simulink model "open_loop"  (R2019a)
settings: Solver=FixedStepAuto  StartTime=0.0  StopTime=10.0  FixedStep=1/100  RelTol=1e-3  AbsTol=1e-3
model workspace: external: MATLAB File params.m (data not in the file)
values from neighbouring files (symbols this model uses):
  An = double(subs(A, [x;ctrl] , [x_lin; u_lin] ))    [linearization.m]
  b = 2.75E-11    (= 2.75e-11)    [linearization.m]    (also in main.m)
  Bn = double(subs(B, [x;ctrl] , [x_lin; u_lin] ))    [linearization.m]
  Cn = eye(size(x,1))    [linearization.m]
  Dn = zeros(size(x,1),4)    [linearization.m]
  g = 9.81    [linearization.m]    (also in main.m)
  k = 1E-9    (= 1e-09)    [linearization.m]    (also in main.m)
  m = 0.027    [linearization.m]    (also in main.m)
  scenario = 1    [main.m]
  u_lin = repmat(0.027*g/4, [4 1])    [main.m]
  x0 = [0 0 0  0 0 0  deg2rad(20) deg2rad(20) deg2rad(0) 0 0 0]'    [main.m]
  x_lin = zeros(12,1)    [main.m]
undefined symbols (not defined in the file or in its folder): sigbuilder_block
libraries: nesl_utility x9
settings Model: Creator=Jocke  LastModifiedBy=lucas
settings SolverCC: AutoScaleAbsTol=off
settings DataIOCC: ReturnWorkspaceOutputs=off
settings DebuggingCC: ArithmeticOperatorsInVariantConditions=warning
settings SFSimCC: SimUseLocalCustomCode=off
settings RTWCC: RTWUseLocalCustomCode=off
settings CodeAppCC: StateflowObjectComments=on
settings SimscapeCC: SimscapeNormalizeSystem=off  SimscapeLogType=all  SimscapeLogDataHistory=10000

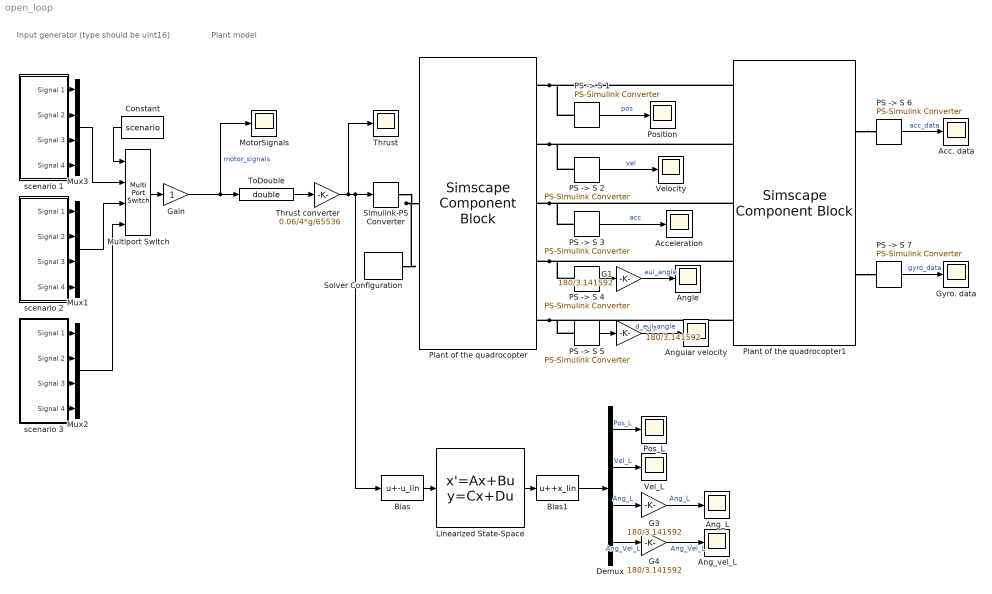
== system open_loop ==
  note: Input generator
      | (type should be uint16)
  note: Plant model
  Acc. data : Scope
  Acceleration : Scope
  Ang_L : Scope
  Ang_vel_L : Scope
  Angle : Scope
  Angular velocity : Scope
  Bias : Bias  Bias=-u_lin
  Bias1 : Bias  Bias=+x_lin
  Constant : Constant  Value=scenario
  Demux : Demux
  G{1..4} (4 alike) : Gain  Gain=180/3.141592
  Gain : Gain
  Gyro. data : Scope
  Linearized State-Space : StateSpace  A=An  B=Bn  C=Cn  D=Dn  InitialCondition=x0
  MotorSignals : Scope
  Multiport Switch : MultiPortSwitch
  Mux1 : Mux
  Mux2 : Mux
  Mux3 : Mux
  PS -> S {1..7} (7 alike) : nesl_utility/PS-Simulink Converter  PhysicalDomain=network_engine_domain  SubClassName=ps_output  LeftPortType=input  RightPortType=output  PseudoPeriodic=off  Frequencies=[]  Unit=1  AffineConversion=off
  Plant of the quadrocopter : SimscapeComponentBlock  SourceFile=plant  ComponentPath=plant  ComponentVariants=plant  ComponentVariantNames=plant  ClassName=plant  SchemaVersion=1  m=m kg  g=g m/s^2  d=d m  k=k s^2*N/rad^2  b=b N*m/(rad/s)^2
      settings: CopyFcn=simscape.engine.sli.internal.componentblockcallback(gcbh,'COPY')  PreCopyFcn=simscape.engine.sli.internal.componentblockcallback(gcbh,'PRECOPY')  PreDeleteFcn=simscape.engine.sli.internal.componentblockcallback(gcbh,'PREDELETE')
      mask Type: Plant of quadrocopter
  Plant of the quadrocopter1 : SimscapeComponentBlock  SourceFile=sensors  ComponentPath=sensors  ComponentVariants=sensors  ComponentVariantNames=sensors  ClassName=sensors  SchemaVersion=1  m=m kg  g=g m/s^2  d=d m  k=k  b=b
      settings: CopyFcn=simscape.engine.sli.internal.componentblockcallback(gcbh,'COPY')  PreCopyFcn=simscape.engine.sli.internal.componentblockcallback(gcbh,'PRECOPY')  PreDeleteFcn=simscape.engine.sli.internal.componentblockcallback(gcbh,'PREDELETE')
      mask Type: Plant of quadrocopter
  Pos_L : Scope
  Position : Scope
  Simulink-PS Converter : nesl_utility/Simulink-PS Converter  PhysicalDomain=network_engine_domain  SubClassName=ps_input  LeftPortType=input  RightPortType=output  PseudoPeriodic=off  Frequencies=[]  NoiseDistribution=none  NoiseParameters=[]  Unit=1  AffineConversion=off  FilteringAndDerivatives=zero  SimscapeFilterOrder=1  InputFilterTimeConstant=0.001  UdotUserProvided=1
  Solver Configuration : nesl_utility/Solver Configuration  PhysicalDomain=network_engine_domain  SubClassName=solver  LeftPortType=input  RightPortType=generic  Tones=[]  Harmonics=[]  SimulateNoise=off  Profile=off  UseLocalSampling=off  EnableSwitchedLinearOptims=on  FrequencyDomain=off  UseCCode=off  RelTol=0.001  AbsTol=1e-06  MinStep=1e-09  ToWorkspace=off  RevertToSquareIcSolve=off  NumHomotopyIterations=100  PhasorMode=off  PhasorModeNumHarmonics=1  DoDC=off  ResidualTolerance=1e-09  UseLocalSolver=off  LocalSolverChoice=NE_BACKWARD_EULER_ADVANCER  LocalSolverSampleTime=0.001  DoFixedCost=off  MaxNonlinIter=3  MaxModeIter=2  LinearAlgebra=Sparse  EquationFormulation=NE_TIME_EF  DelaysMemoryBudget=1024  AutomaticFiltering=on  FilteringTimeConstant=0.001  PartitionStorageMethod=AS_NEEDED  PartitionMemoryBudget=1024  PartitionMethod=FAST
  Thrust : Scope
  Thrust converter : Gain  Gain=0.06/4*g/65536
  ToDouble : DataTypeConversion  OutDataTypeStr=double  RndMeth=Round  SaturateOnIntegerOverflow=on
  Vel_L : Scope
  Velocity : Scope
  scenario 1 : Subsystem  Tag=STV Subsys  LoadFcn=sigbuilder_block('load');  StartFcn=sigbuilder_block('start');  StopFcn=sigbuilder_block('stop');  ClipboardFcn=sigbuilder_block('clipboard');  mask(Sigbuilder block){tuvar=[0:10]}
      mask help: Simulink:masks:SigbuilderBlock_MD
      mask init:
      | if ~strcmp(get_param(bdroot(gcbh),'SimulationStatus'),'stopped') tuvar = sigbuilder_block('maskInit'); end
      settings: CopyFcn=sigbuilder_block('copy');  DeleteFcn=sigbuilder_block('delete');  ModelCloseFcn=sigbuilder_block('modelClose');  PreSaveFcn=sigbuilder_block('preSave');  PauseFcn=sigbuilder_block('pause');  ContinueFcn=sigbuilder_block('continue');  NameChangeFcn=sigbuilder_block('namechange');  OpenFcn=sigbuilder_block('open',[382.5 57 795 560.25 ]);  CloseFcn=sigbuilder_block('close');
      mask Display: plot(0, 0, 100, 100,[2, 2, 32, 32, 2], [68, 8, 8, 68, 68],[32, 2], [38, 38], [32, 19, 2],[53, 60, 44], [32, 17, 17, 2],[16, 16, 31, 31]);txt = getActiveGroup(gcbh);text(2, 100, txt,'verticalAlignment', 'top');
  scenario 2 : Subsystem  Tag=STV Subsys  LoadFcn=sigbuilder_block('load');  StartFcn=sigbuilder_block('start');  StopFcn=sigbuilder_block('stop');  ClipboardFcn=sigbuilder_block('clipboard');  mask(Sigbuilder block){tuvar=[0:10]}
      mask help: Simulink:masks:SigbuilderBlock_MD
      mask init:
      | if ~strcmp(get_param(bdroot(gcbh),'SimulationStatus'),'stopped') tuvar = sigbuilder_block('maskInit'); end
      settings: CopyFcn=sigbuilder_block('copy');  DeleteFcn=sigbuilder_block('delete');  ModelCloseFcn=sigbuilder_block('modelClose');  PreSaveFcn=sigbuilder_block('preSave');  PauseFcn=sigbuilder_block('pause');  ContinueFcn=sigbuilder_block('continue');  NameChangeFcn=sigbuilder_block('namechange');  OpenFcn=sigbuilder_block('open',[378.75 53.25 795 560.25 ]);  CloseFcn=sigbuilder_block('close');
      mask Display: plot(0, 0, 100, 100,[2, 2, 32, 32, 2], [68, 8, 8, 68, 68],[32, 2], [38, 38], [32, 19, 2],[53, 60, 44], [32, 17, 17, 2],[16, 16, 31, 31]);txt = getActiveGroup(gcbh);text(2, 100, txt,'verticalAlignment', 'top');
  scenario 3 : Subsystem  Tag=STV Subsys  LoadFcn=sigbuilder_block('load');  StartFcn=sigbuilder_block('start');  StopFcn=sigbuilder_block('stop');  ClipboardFcn=sigbuilder_block('clipboard');  mask(Sigbuilder block){tuvar=[0:10]}
      mask help: Simulink:masks:SigbuilderBlock_MD
      mask init:
      | if ~strcmp(get_param(bdroot(gcbh),'SimulationStatus'),'stopped') tuvar = sigbuilder_block('maskInit'); end
      settings: CopyFcn=sigbuilder_block('copy');  DeleteFcn=sigbuilder_block('delete');  ModelCloseFcn=sigbuilder_block('modelClose');  PreSaveFcn=sigbuilder_block('preSave');  PauseFcn=sigbuilder_block('pause');  ContinueFcn=sigbuilder_block('continue');  NameChangeFcn=sigbuilder_block('namechange');  OpenFcn=sigbuilder_block('open',[285.75 75.75 817.5 560.25 ]);  CloseFcn=sigbuilder_block('close');
      mask Display: plot(0, 0, 100, 100,[2, 2, 32, 32, 2], [68, 8, 8, 68, 68],[32, 2], [38, 38], [32, 19, 2],[53, 60, 44], [32, 17, 17, 2],[16, 16, 31, 31]);txt = getActiveGroup(gcbh);text(2, 100, txt,'verticalAlignment', 'top');
  wires:
  "PS -> S 7"/1 -> Gyro. data/1  "gyro_data"
  "PS -> S 6"/1 -> Acc. data/1  "acc_data"
  Multiport Switch/1 -> Gain/1
  G1/1 -> Angle/1  "eul_angle"
  G2/1 -> Angular velocity/1  "d_eul_angle"
  ToDouble/1 -> Thrust converter/1
  Thrust converter/1 -> Bias/1, Simulink-PS Converter/1, Thrust/1
  "PS -> S 1"/1 -> Position/1  "pos"
  "PS -> S 5"/1 -> G2/1
  "PS -> S 4"/1 -> G1/1
  "PS -> S 3"/1 -> Acceleration/1  "acc"
  "PS -> S 2"/1 -> Velocity/1  "vel"
  scenario 1/2(Signal 2) -> Mux3/2
  scenario 1/1(Signal 1) -> Mux3/1
  scenario 1/3(Signal 3) -> Mux3/3
  scenario 1/4(Signal 4) -> Mux3/4
  scenario 2/3(Signal 3) -> Mux1/3
  scenario 2/4(Signal 4) -> Mux1/4
  scenario 2/2(Signal 2) -> Mux1/2
  Mux1/1 -> Multiport Switch/3
  scenario 2/1(Signal 1) -> Mux1/1
  Mux3/1 -> Multiport Switch/2
  Gain/1 -> MotorSignals/1, ToDouble/1  "motor_signals"
  scenario 3/3(Signal 3) -> Mux2/3
  scenario 3/4(Signal 4) -> Mux2/4
  scenario 3/2(Signal 2) -> Mux2/2
  scenario 3/1(Signal 1) -> Mux2/1
  Mux2/1 -> Multiport Switch/4
  Constant/1 -> Multiport Switch/1
  Linearized State-Space/1 -> Bias1/1
  Demux/1 -> Pos_L/1  "Pos_L"
  Demux/2 -> Vel_L/1  "Vel_L"
  Bias/1 -> Linearized State-Space/1
  Bias1/1 -> Demux/1
  G3/1 -> Ang_L/1  "Ang_L"
  Demux/3 -> G3/1  "Ang_L"
  G4/1 -> Ang_vel_L/1  "Ang_Vel_L"
  Demux/4 -> G4/1  "Ang_Vel_L"
  connections:
  Plant of the quadrocopter/LConn1 -- Solver Configuration/RConn1 -- Simulink-PS Converter/RConn1
  Plant of the quadrocopter/RConn1 -- "PS -> S 1"/LConn1 -- Plant of the quadrocopter1/LConn1
  Plant of the quadrocopter/RConn2 -- "PS -> S 2"/LConn1 -- Plant of the quadrocopter1/LConn2
  Plant of the quadrocopter/RConn3 -- "PS -> S 3"/LConn1 -- Plant of the quadrocopter1/LConn3
  Plant of the quadrocopter/RConn4 -- "PS -> S 4"/LConn1 -- Plant of the quadrocopter1/LConn4
  Plant of the quadrocopter/RConn5 -- "PS -> S 5"/LConn1 -- Plant of the quadrocopter1/LConn5
  Plant of the quadrocopter1/RConn1 -- "PS -> S 6"/LConn1
  Plant of the quadrocopter1/RConn2 -- "PS -> S 7"/LConn1

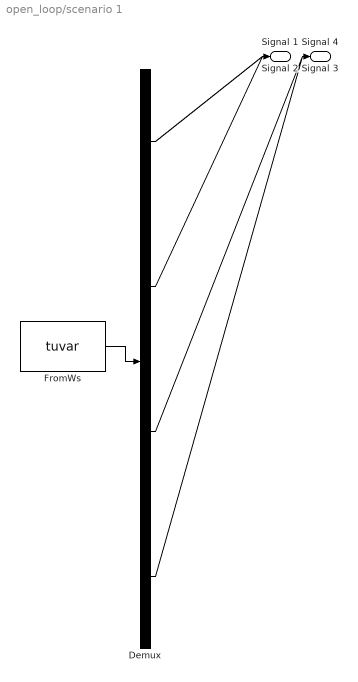
== system open_loop/scenario 1 ==
  Demux : Demux  Tag=STV Demux
  FromWs : FromWorkspace  Tag=STV FromWs  VariableName=tuvar  SampleTime=0
      SigBuilderData=|
      | common.afterFinalStr = 'Extrapolate'
      | common.sampleTime = 0
      | dataSet.timeRange = [0 10]
      | dataSet.name = 'Motors_scen_1'
      | sbobj.Groups.Name = 'Motors_scen_1'
      | sbobj.Groups.Signals(1).Name = 'Signal 1'
      | sbobj.Groups.Signals(1).XData = [0 4 4 10]
      | sbobj.Groups.Signals(1).YData = [-1.94289029309e-16 -1.94289029309e-16 10 10]
      | sbobj.Groups.Signals(2).Name = 'Signal 2'
      | sbobj.Groups.Signals(2).XData = [0 4 4 10]
      | sbobj.Groups.Signals(2).YData = [0 0 10 10]
      | sbobj.Groups.Signals(3).Name = 'Signal 3'
      | sbobj.Groups.Signals(3).XData = [0 10]
      | sbobj.Groups.Signals(3).YData = [0 0]
      | sbobj.Groups.Signals(4).Name = 'Signal 4'
      | sbobj.Groups.Signals(4).XData = [0 5.04 10]
      | sbobj.Groups.Signals(4).YData = [0 0 0]
  Signal 1 : Outport  Tag=STV Outport
  Signal 2 : Outport  Tag=STV Outport  Port=2
  Signal 3 : Outport  Tag=STV Outport  Port=3
  Signal 4 : Outport  Tag=STV Outport  Port=4
  wires:
  FromWs/1 -> Demux/1
  Demux/1 -> Signal 1/1
  Demux/2 -> Signal 2/1
  Demux/3 -> Signal 3/1
  Demux/4 -> Signal 4/1

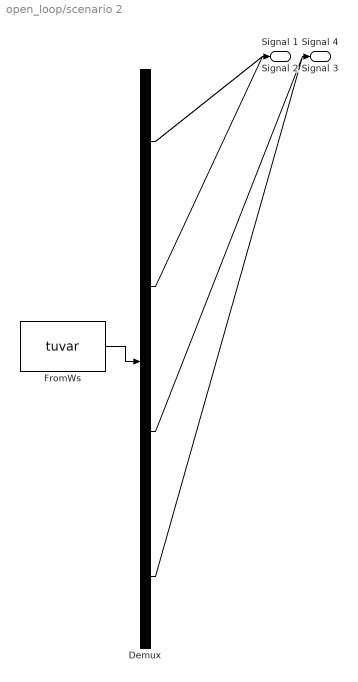
== system open_loop/scenario 2 ==
  Demux : Demux  Tag=STV Demux
  FromWs : FromWorkspace  Tag=STV FromWs  VariableName=tuvar  SampleTime=0
      SigBuilderData=|
      | common.afterFinalStr = 'Extrapolate'
      | common.sampleTime = 0
      | dataSet.timeRange = [0 10]
      | dataSet.name = 'Motors_scen_1'
      | sbobj.Groups.Name = 'Motors_scen_1'
      | sbobj.Groups.Signals(1).Name = 'Signal 1'
      | sbobj.Groups.Signals(1).XData = [0 4 4 10]
      | sbobj.Groups.Signals(1).YData = [-1.94289029309e-16 -1.94289029309e-16 1000 1000]
      | sbobj.Groups.Signals(2).Name = 'Signal 2'
      | sbobj.Groups.Signals(2).XData = [0 10]
      | sbobj.Groups.Signals(2).YData = [0 0]
      | sbobj.Groups.Signals(3).Name = 'Signal 3'
      | sbobj.Groups.Signals(3).XData = [0 6 6 10]
      | sbobj.Groups.Signals(3).YData = [0 0 2000 2000]
      | sbobj.Groups.Signals(4).Name = 'Signal 4'
      | sbobj.Groups.Signals(4).XData = [0 5.04 10]
      | sbobj.Groups.Signals(4).YData = [0 0 0]
  Signal 1 : Outport  Tag=STV Outport
  Signal 2 : Outport  Tag=STV Outport  Port=2
  Signal 3 : Outport  Tag=STV Outport  Port=3
  Signal 4 : Outport  Tag=STV Outport  Port=4
  wires:
  FromWs/1 -> Demux/1
  Demux/1 -> Signal 1/1
  Demux/2 -> Signal 2/1
  Demux/3 -> Signal 3/1
  Demux/4 -> Signal 4/1

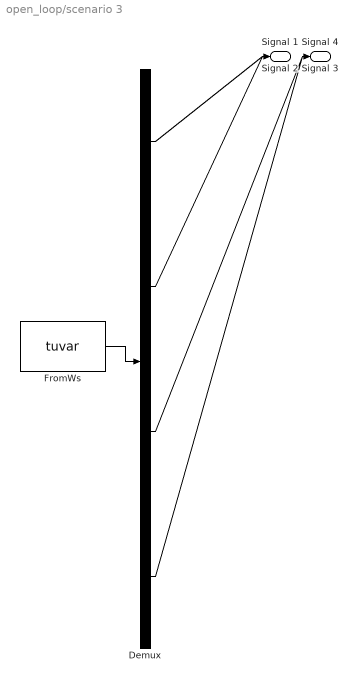
== system open_loop/scenario 3 ==
  Demux : Demux  Tag=STV Demux
  FromWs : FromWorkspace  Tag=STV FromWs  VariableName=tuvar  SampleTime=0
      SigBuilderData=|
      | common.afterFinalStr = 'Extrapolate'
      | common.sampleTime = 0
      | dataSet.timeRange = [0 10]
      | dataSet.name = 'Motors_scen_1'
      | sbobj.Groups.Name = 'Motors_scen_1'
      | sbobj.Groups.Signals(1).Name = 'Signal 1'
      | sbobj.Groups.Signals(1).XData = [0 10]
      | sbobj.Groups.Signals(1).YData = [500 500]
      | sbobj.Groups.Signals(2).Name = 'Signal 2'
      | sbobj.Groups.Signals(2).XData = [0 10]
      | sbobj.Groups.Signals(2).YData = [1000 1000]
      | sbobj.Groups.Signals(3).Name = 'Signal 3'
      | sbobj.Groups.Signals(3).XData = [0 10]
      | sbobj.Groups.Signals(3).YData = [500 500]
      | sbobj.Groups.Signals(4).Name = 'Signal 4'
      | sbobj.Groups.Signals(4).XData = [0 10]
      | sbobj.Groups.Signals(4).YData = [1000 1000]
  Signal 1 : Outport  Tag=STV Outport
  Signal 2 : Outport  Tag=STV Outport  Port=2
  Signal 3 : Outport  Tag=STV Outport  Port=3
  Signal 4 : Outport  Tag=STV Outport  Port=4
  wires:
  FromWs/1 -> Demux/1
  Demux/1 -> Signal 1/1
  Demux/2 -> Signal 2/1
  Demux/3 -> Signal 3/1
  Demux/4 -> Signal 4/1
